simulink model "sistema1"  (R2023a)
settings: Solver=VariableStepAuto  StartTime=0.0  StopTime=100.00  RelTol=1e-3
settings Model: Creator=belen  LastModifiedBy=belen
settings DataIOCC: ReturnWorkspaceOutputs=off  TimeSaveName=t

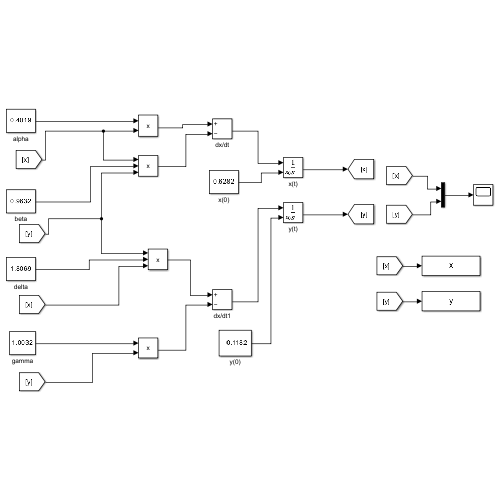
[thumbnail: Simulink's stored preview of the top-level diagram]
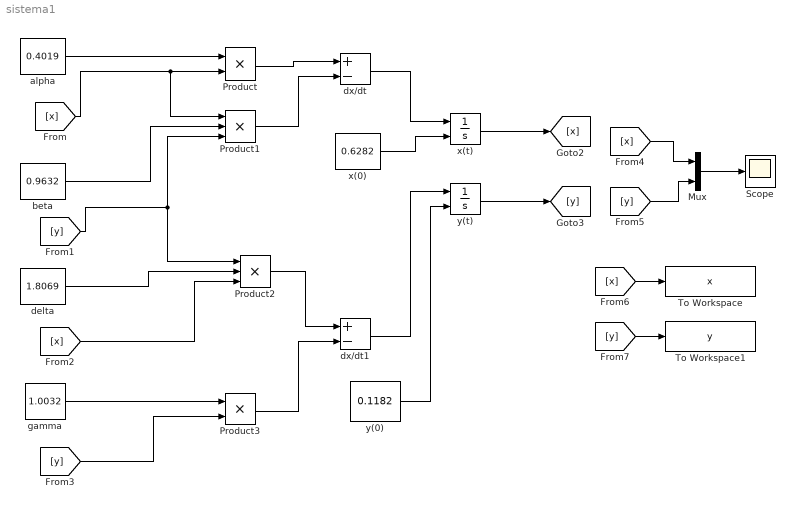
== system sistema1 ==
  Mux : Mux  Inputs=2
  Product : Product
  Product1 : Product  Inputs=3
  Product2 : Product  Inputs=3
  Product3 : Product
  Scope : Scope
  To Workspace : ToWorkspace  VariableName=x  SampleTime=-1
  To Workspace1 : ToWorkspace  VariableName=y  SampleTime=-1
  alpha : Constant  Value=0.4019
  beta : Constant  Value=0.9632
  delta : Constant  Value=1.8069
  dx/dt : Sum  Inputs=+-
  dx/dt1 : Sum  Inputs=+-
  gamma : Constant  Value=1.0032
  x(0) : Constant  Value=0.6282
  x(t) : Integrator  InitialConditionSource=external
  y(0) : Constant  Value=0.1182
  y(t) : Integrator  InitialConditionSource=external
  wires:
  x(t)/1 -> [x]
  y(t)/1 -> [y]
  Mux/1 -> Scope/1
  [x] -> Mux/1
  [y] -> Mux/2
  [x] -> Product/2, Product1/1
  beta/1 -> Product1/2
  [y] -> Product2/1, Product1/3
  delta/1 -> Product2/2
  [x] -> Product2/3
  gamma/1 -> Product3/1
  [y] -> Product3/2
  Product2/1 -> dx/dt1/1
  Product3/1 -> dx/dt1/2
  Product/1 -> dx/dt/1
  Product1/1 -> dx/dt/2
  dx/dt/1 -> x(t)/1
  dx/dt1/1 -> y(t)/1
  y(0)/1 -> y(t)/2
  x(0)/1 -> x(t)/2
  alpha/1 -> Product/1
  [y] -> To Workspace1/1
  [x] -> To Workspace/1
